simulink model "non_linear_system"  (R2020b)
settings: Solver=FixedStepAuto  StartTime=0.0  StopTime=100  FixedStep=0.001  RelTol=1e-3
values from neighbouring files (symbols this model uses):
  A = double(subs(A, [x; u], [x_equ; u_equ]))    [Second_order_perturbation.m]    (also in main.m)
  amp = 0.3    [Second_order_perturbation.m]    (also in main.m)
  B = double(subs(B, [x; u], [x_equ; u_equ]))    [Second_order_perturbation.m]    (also in main.m)
  u_equ = 0.16    [Second_order_perturbation.m]    (also in main.m)
  x_equ = [0.2; 0]    [Second_order_perturbation.m]    (also in main.m)
settings Model: Creator=soren  LastModifiedBy=soren

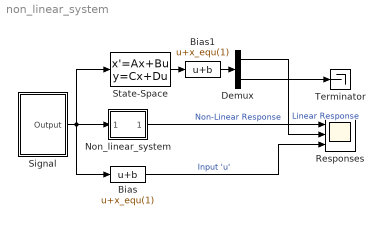
== system non_linear_system ==
  Bias : Bias  Bias=x_equ(1)
  Bias1 : Bias  Bias=x_equ(1)
  Demux : Demux  Outputs=2
  Non_linear_system : Subsystem
  Responses : Scope  NumInputPorts=3
  Signal : Subsystem
  State-Space : StateSpace  A=A  B=B  C=eye(2,2)  D=zeros(2,1)  InitialCondition=0
  Terminator : Terminator
  wires:
  Non_linear_system/1(Output) -> Responses/1  "Non-Linear Response"
  Signal/1(Output) -> Non_linear_system/1(Input), State-Space/1, Bias/1
  State-Space/1 -> Bias1/1
  Bias1/1 -> Demux/1
  Demux/1 -> Responses/2  "Linear Response"
  Bias/1 -> Responses/3  "Input 'u'"
  Demux/2 -> Terminator/1

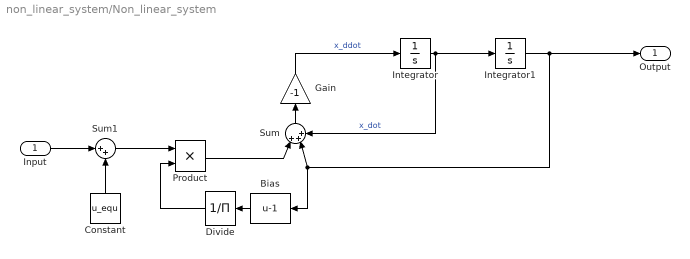
== system non_linear_system/Non_linear_system ==
  Input : Inport
  Bias : Bias  Bias=-1
  Constant : Constant  Value=u_equ
  Divide : Product  Inputs=/
  Gain : Gain  Gain=-1
  Integrator : Integrator
  Integrator1 : Integrator  InitialCondition=x_equ(1)
  Product : Product
  Sum : Sum  Inputs=|+++
  Sum1 : Sum  Inputs=|++
  Output : Outport
  wires:
  Integrator/1 -> Sum/3, Integrator1/1  "x_dot"
  Gain/1 -> Integrator/1  "x_ddot"
  Constant/1 -> Sum1/2
  Input/1 -> Sum1/1
  Integrator1/1 -> Output/1, Bias/1, Sum/2
  Bias/1 -> Divide/1
  Sum/1 -> Gain/1
  Sum1/1 -> Product/1
  Product/1 -> Sum/1
  Divide/1 -> Product/2

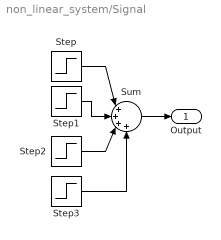
== system non_linear_system/Signal ==
  Step : Step  Time=20  After=0.16*amp  SampleTime=0
  Step1 : Step  Time=40  After=-0.16*amp  SampleTime=0
  Step2 : Step  Time=60  After=-0.16*amp  SampleTime=0
  Step3 : Step  Time=80  After=0.16*amp  SampleTime=0
  Sum : Sum  Inputs=|++++
  Output : Outport
  wires:
  Sum/1 -> Output/1
  Step2/1 -> Sum/3
  Step/1 -> Sum/1
  Step1/1 -> Sum/2
  Step3/1 -> Sum/4
